simulink subsystem "HEVMM"  (R2023b)
settings: Solver=VariableStepAuto  StartTime=0.0  StopTime=10.0  RelTol=1e-3
undefined symbols (not defined in the file): PlntHevMmCltchPrs, PlntHevMmEngDamp, PlntHevMmEngInertia, PlntHevMmGenGearRatio, PlntHevMmMotGearRatio
libraries: autolibcoupling x3, autolibsharedcoupling x3
settings Model: ModifiedByFormat=The MathWorks, Inc.  Creator=The MathWorks, Inc.  LastModifiedBy=The MathWorks, Inc.
settings SolverCC: MaxZcPerStep=1
settings DebuggingCC: UnconnectedInputMsg=warning  UnconnectedOutputMsg=warning  UnconnectedLineMsg=warning  SubsystemReferenceDiagnosticForUnitTest=warning
settings ModelReferenceCC: EnableRefExpFcnMdlSchedulingChecks=on
settings RTWCC: DLArmComputeVersion=19.05

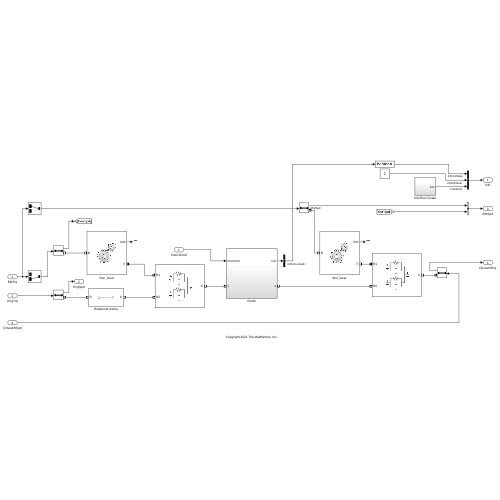
[thumbnail: Simulink's stored preview of the top-level diagram]
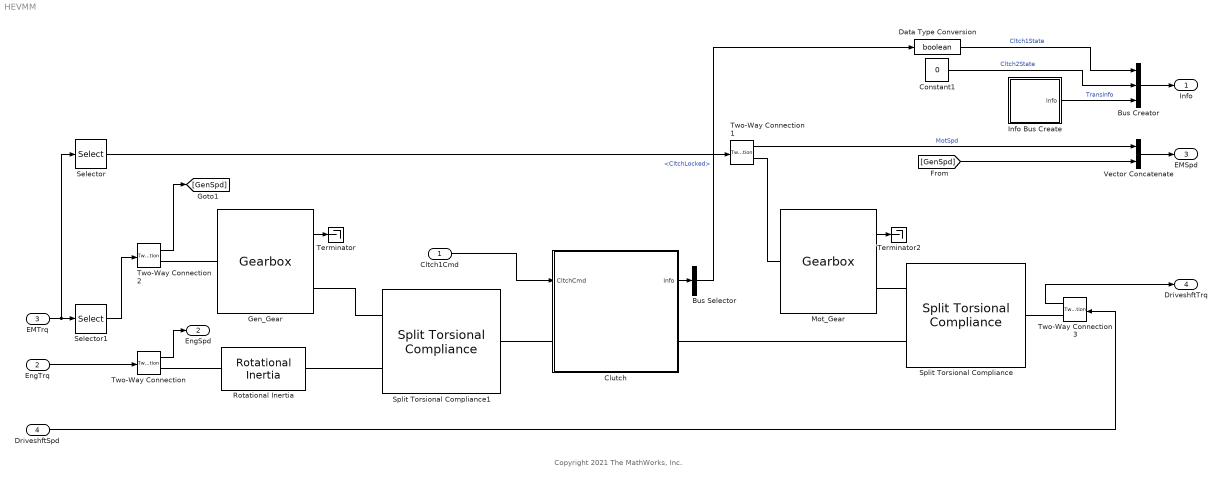
== system HEVMM ==
  note: Copyright 2021 The MathWorks, Inc.
  Cltch1Cmd : Inport
  EngTrq : Inport  Port=2
  EMTrq : Inport  Port=3
  DriveshftSpd : Inport  Port=4
  Bus Creator : BusCreator  Inputs=3
  Bus Selector : BusSelector  OutputSignals=Cltch.CltchLocked
  Clutch : Subsystem
  Constant1 : Constant  Value=0  SampleTime=-1
  Data Type Conversion : DataTypeConversion  OutDataTypeStr=boolean  SaturateOnIntegerOverflow=off  RndMeth=Floor
  Gen_Gear : autolibcoupling/Gearbox  port_config=Two-way connection  input_config=Torque input - velocity output  DiffEffModelPopup=Constant  InterpMethod=Flat  dirSwitch=on  extTamb=off  N=PlntHevMmGenGearRatio  J1=PlntHevMmGenGearInInertia  J2=PlntHevMmGenGearOutInertia  b1=PlntHevMmGenGearInDamp  b2=PlntHevMmGenGearOutDamp  theta1_o=0  w1_o=PlntHevMmGenGearInitVel  eta=PlntHevMmGenGearEff  eta_tbl=reshape([0.64 0.76 0.8 0.81 0.83 0.84 0.84 0.56 0.73 0.78 0.8 0.83 0.84 0.84 0.54 0.71 0.77 0.8 0.82 0.84 0.84 0.53 0.71 0.77 0.8 0.83 0.84 0.84 0.51 0.71 0.77 0.8 0.83 0.84 0.85 0.52 0.7 0.77 0.8 0.83 0.84 0.85 0.51 0.71 0.76 0.79 0.83 0.84 0.85 0.5 0.69 0.76 0.79 0.82 0.84 0.85 0.45 0.68 0.75 0.78 0.82 0.84 0.85 0.43 0.67 0.74 0.78 0.81 0.83 0.84 0.38 0.63 0.71 0.75 0.8 0.82 0.83 0.81 0.86 0.88 0.89 0.89 0.89 0.9 0.77 0.85 0.87 0.88 0.89 0.9 0.9 0.72 0.82 0.86 0.87 0.88 0.89 0.9 0.68 0.8 0.84 0.86 0.88 0.89 0.89 0.67 0.8 0.84 0.86 0.88 0.89 0.9 0.67 0.8 0.84 0.86 0.88 0.89 0.9 0.65 0.8 0.84 0.86 0.88 0.89 0.9 0.64 0.79 0.83 0.86 0.88 0.89 0.9 0.63 0.78 0.83 0.86 0.88 0.89 0.9 0.59 0.76 0.82 0.85 0.87 0.89 0.9 0.53 0.73 0.8 0.83 0.86 0.88 0.89], 7, 11, 2)  Trq_bpts=[25, 50, 75, 100, 150, 200, 250]  omega_bpts=[52.4 78.5 105 131 157 183 209 262 314 419 524]  Temp_bpts=[290 358]  Tamb=297.15  blkID=0
  Info Bus Create : Subsystem
  Mot_Gear : autolibcoupling/Gearbox  port_config=Two-way connection  input_config=Torque input - velocity output  DiffEffModelPopup=Constant  InterpMethod=Flat  dirSwitch=on  extTamb=off  N=PlntHevMmMotGearRatio  J1=PlntHevMmMotGearInInertia  J2=PlntHevMmMotGearOutInertia  b1=PlntHevMmMotGearInDamp  b2=PlntHevMmMotGearOutDamp  theta1_o=0  w1_o=PlntHevMmMotGearInitVel  eta=PlntHevMmMotGearEff  eta_tbl=reshape([0.64 0.76 0.8 0.81 0.83 0.84 0.84 0.56 0.73 0.78 0.8 0.83 0.84 0.84 0.54 0.71 0.77 0.8 0.82 0.84 0.84 0.53 0.71 0.77 0.8 0.83 0.84 0.84 0.51 0.71 0.77 0.8 0.83 0.84 0.85 0.52 0.7 0.77 0.8 0.83 0.84 0.85 0.51 0.71 0.76 0.79 0.83 0.84 0.85 0.5 0.69 0.76 0.79 0.82 0.84 0.85 0.45 0.68 0.75 0.78 0.82 0.84 0.85 0.43 0.67 0.74 0.78 0.81 0.83 0.84 0.38 0.63 0.71 0.75 0.8 0.82 0.83 0.81 0.86 0.88 0.89 0.89 0.89 0.9 0.77 0.85 0.87 0.88 0.89 0.9 0.9 0.72 0.82 0.86 0.87 0.88 0.89 0.9 0.68 0.8 0.84 0.86 0.88 0.89 0.89 0.67 0.8 0.84 0.86 0.88 0.89 0.9 0.67 0.8 0.84 0.86 0.88 0.89 0.9 0.65 0.8 0.84 0.86 0.88 0.89 0.9 0.64 0.79 0.83 0.86 0.88 0.89 0.9 0.63 0.78 0.83 0.86 0.88 0.89 0.9 0.59 0.76 0.82 0.85 0.87 0.89 0.9 0.53 0.73 0.8 0.83 0.86 0.88 0.89], 7, 11, 2)  Trq_bpts=[25, 50, 75, 100, 150, 200, 250]  omega_bpts=[52.4 78.5 105 131 157 183 209 262 314 419 524]  Temp_bpts=[290 358]  Tamb=297.15  blkID=0
  Rotational Inertia : autolibsharedcoupling/Rotational Inertia  port_config=Two-way connection  extInfo=off  externJ=off  J=PlntHevMmEngInertia  b=PlntHevMmEngDamp  omega_o=PlntHevMmEngInitVel  blkID=0  aMode=1
      settings: LibrarySourceBlock=autolibcoupling/Rotational Inertia
  Selector : Selector  InputPortWidth=2  IndexOptions=Index vector (dialog)  Indices=[1]  OutputSizes=1
  Selector1 : Selector  InputPortWidth=2  IndexOptions=Index vector (dialog)  Indices=[2]  OutputSizes=1
  Split Torsional Compliance : autolibsharedcoupling/Split Torsional Compliance  port_config=Two-way connection  cplrMode=Shaft merge  extInfo=off  k1=PlntDriveshftStiff  b1=PlntDriveshftDamp  omega1_c=PlntDriveshftDampCutoffFreq  theta1_o=0  domega1_o=0  k2=PlntDriveshftStiff  b2=PlntDriveshftDamp  omega2_c=PlntDriveshftDampCutoffFreq  theta2_o=0  domega2_o=0  blkID=0  aMode=1
      settings: LibrarySourceBlock=autolibcoupling/Split Torsional Compliance
  Split Torsional Compliance1 : autolibsharedcoupling/Split Torsional Compliance  port_config=Two-way connection  cplrMode=Shaft merge  extInfo=off  k1=PlntDriveshftStiff  b1=PlntDriveshftDamp  omega1_c=PlntDriveshftDampCutoffFreq  theta1_o=0  domega1_o=0  k2=PlntDriveshftStiff  b2=PlntDriveshftDamp  omega2_c=PlntDriveshftDampCutoffFreq  theta2_o=0  domega2_o=0  blkID=0  aMode=1
      settings: LibrarySourceBlock=autolibcoupling/Split Torsional Compliance
  Terminator : Terminator
  Terminator2 : Terminator
  Two-Way Connection{,1..3} (4 alike) : TwoWayConnection
  Vector Concatenate : Concatenate
  Info : Outport  VectorParamsAs1DForOutWhenUnconnected=off  BusOutputAsStruct=on
  EngSpd : Outport  Port=2  VectorParamsAs1DForOutWhenUnconnected=off  BusOutputAsStruct=on
  EMSpd : Outport  Port=3  VectorParamsAs1DForOutWhenUnconnected=off  BusOutputAsStruct=on
  DriveshftTrq : Outport  Port=4  VectorParamsAs1DForOutWhenUnconnected=off
  wires:
  Bus Selector/1 -> Data Type Conversion/1  "<CltchLocked>"
  Mot_Gear/1 -> Terminator2/1
  Two-Way Connection1/1 -> Vector Concatenate/1  "MotSpd"
  Clutch/1(Info) -> Bus Selector/1
  EMTrq/1 -> Selector1/1, Selector/1
  EngTrq/1 -> Two-Way Connection/1
  Cltch1Cmd/1 -> Clutch/1(CltchCmd)
  Gen_Gear/1 -> Terminator/1
  Selector/1 -> Two-Way Connection1/1
  Two-Way Connection/1 -> EngSpd/1
  Vector Concatenate/1 -> EMSpd/1
  [GenSpd] -> Vector Concatenate/2
  Bus Creator/1 -> Info/1
  Constant1/1 -> Bus Creator/2  "Cltch2State"
  Info Bus Create/1(Info) -> Bus Creator/3  "TransInfo"
  DriveshftSpd/1 -> Two-Way Connection3/1
  Two-Way Connection3/1 -> DriveshftTrq/1
  Data Type Conversion/1 -> Bus Creator/1  "Cltch1State"
  Selector1/1 -> Two-Way Connection2/1
  Two-Way Connection2/1 -> [GenSpd]
  connections:
  Two-Way Connection1/RConn1 -- Mot_Gear/LConn1
  Mot_Gear/RConn1 -- Split Torsional Compliance/LConn1
  Clutch/RConn1 -- Split Torsional Compliance/LConn2
  Two-Way Connection3/RConn1 -- Split Torsional Compliance/RConn1
  Two-Way Connection2/RConn1 -- Gen_Gear/LConn1
  Split Torsional Compliance1/RConn1 -- Clutch/LConn1
  Gen_Gear/RConn1 -- Split Torsional Compliance1/LConn1
  Rotational Inertia/RConn1 -- Split Torsional Compliance1/LConn2
  Rotational Inertia/LConn1 -- Two-Way Connection/RConn1

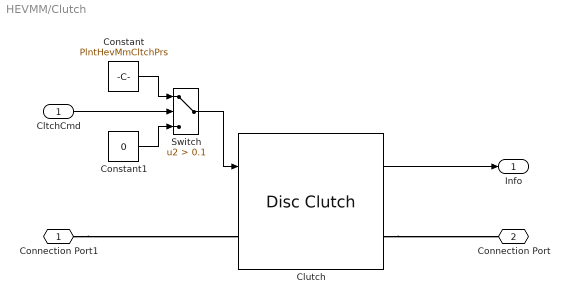
== system HEVMM/Clutch ==
  CltchCmd : Inport
  Clutch : autolibcoupling/Disc Clutch  port_config=Two-way connection  Reff=PlntCltch1Radius  Ndisk=PlntCltch1NumDisk  Aeff=PlntCltch1AppPrsArea  Peng=PlntCltch1EngdPrs  Jin=PlntHevMmCltchInInertia  Jout=PlntCltch1OutInertia  muk=PlntCltch1KinFric  mus=PlntCltch1StatFric  bin=PlntCltch1InDamp  bout=PlntCltch1OutDamp  win_o=PlntCltch1InitInVel  wout_o=PlntCltch1InitOutVel  tauC=PlntHevMmCltchTimeCnst  InitiallyLocked=off  maxAbsSpd=3000  blkID=1
  Constant : Constant  Value=PlntHevMmCltchPrs  SampleTime=-1
  Constant1 : Constant  Value=0
  Switch : Switch  Criteria=u2 > Threshold  Threshold=0.1  SaturateOnIntegerOverflow=off  InputSameDT=off
  Connection Port1 : PMIOPort  Side=Left
  Connection Port : PMIOPort  Port=2  Side=Right
  Info : Outport  VectorParamsAs1DForOutWhenUnconnected=off
  wires:
  Switch/1 -> Clutch/1
  Clutch/1 -> Info/1
  Constant1/1 -> Switch/3
  CltchCmd/1 -> Switch/2
  Constant/1 -> Switch/1
  connections:
  Connection Port1/RConn1 -- Clutch/LConn1
  Clutch/RConn1 -- Connection Port/RConn1

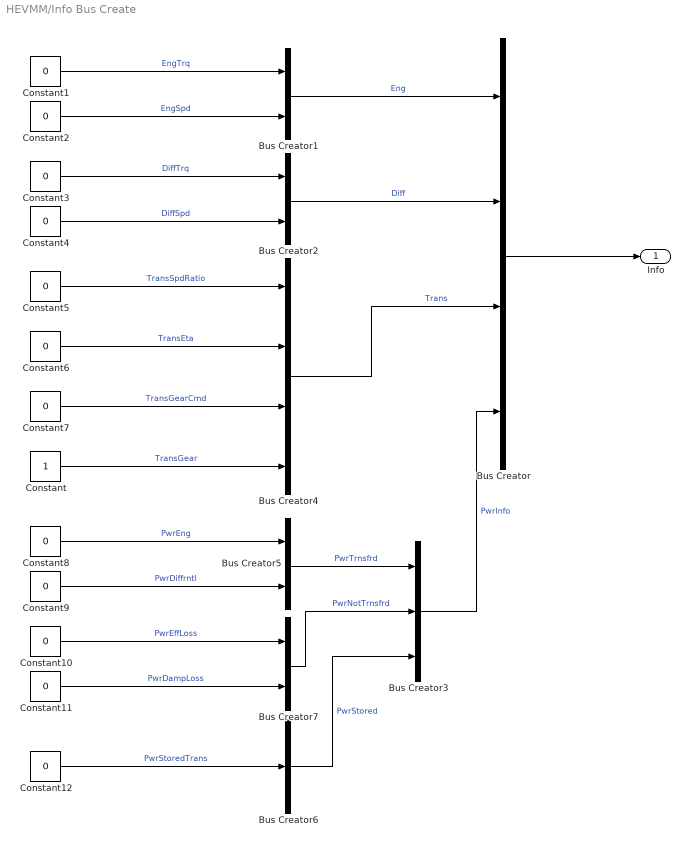
== system HEVMM/Info Bus Create ==
  Bus Creator : BusCreator  Inputs=4
  Bus Creator{1..2,5,7} (4 alike) : BusCreator  Inputs=2
  Bus Creator3 : BusCreator  Inputs=3
  Bus Creator4 : BusCreator  Inputs=4
  Bus Creator6 : BusCreator  Inputs=1
  Constant : Constant  SampleTime=-1
  Constant{1..12} (12 alike) : Constant  Value=0  SampleTime=-1
  Info : Outport
  wires:
  Bus Creator5/1 -> Bus Creator3/1  "PwrTrnsfrd"
  Bus Creator6/1 -> Bus Creator3/3  "PwrStored"
  Bus Creator7/1 -> Bus Creator3/2  "PwrNotTrnsfrd"
  Constant12/1 -> Bus Creator6/1  "PwrStoredTrans"
  Bus Creator2/1 -> Bus Creator/2  "Diff"
  Constant9/1 -> Bus Creator5/2  "PwrDiffrntl"
  Constant7/1 -> Bus Creator4/3  "TransGearCmd"
  Constant10/1 -> Bus Creator7/1  "PwrEffLoss"
  Constant1/1 -> Bus Creator1/1  "EngTrq"
  Constant5/1 -> Bus Creator4/1  "TransSpdRatio"
  Bus Creator/1 -> Info/1
  Constant3/1 -> Bus Creator2/1  "DiffTrq"
  Constant11/1 -> Bus Creator7/2  "PwrDampLoss"
  Constant/1 -> Bus Creator4/4  "TransGear"
  Constant2/1 -> Bus Creator1/2  "EngSpd"
  Bus Creator1/1 -> Bus Creator/1  "Eng"
  Constant6/1 -> Bus Creator4/2  "TransEta"
  Constant4/1 -> Bus Creator2/2  "DiffSpd"
  Constant8/1 -> Bus Creator5/1  "PwrEng"
  Bus Creator3/1 -> Bus Creator/4  "PwrInfo"
  Bus Creator4/1 -> Bus Creator/3  "Trans"
